simulink model "CurrentSource"  (R2024a)
settings: Solver=VariableStepAuto  StartTime=0.0  StopTime=10.0  RelTol=1e-3
undefined symbols (not defined in the file): b, R_B, Rsense, Vdd, Vpp, Vref
settings Model: Creator=Perij  LastModifiedBy=Perij

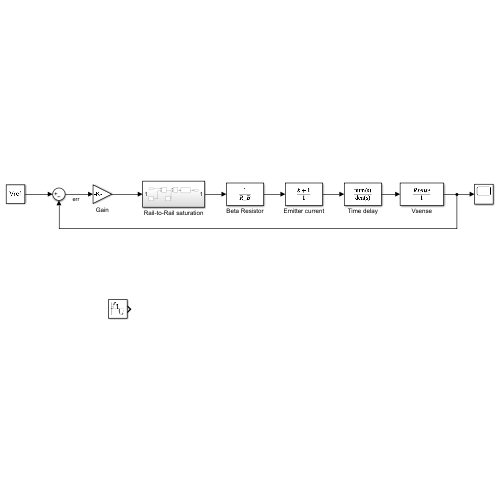
[thumbnail: Simulink's stored preview of the top-level diagram]
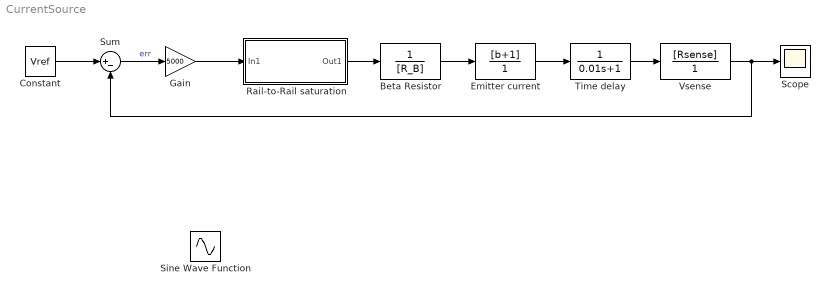
== system CurrentSource ==
  Beta Resistor : TransferFcn  Denominator=[R_B]
  Constant : Constant  Value=Vref
  Emitter current : TransferFcn  Numerator=[b+1]  Denominator=[1]
  Gain : Gain  Gain=5000
  Rail-to-Rail saturation : Subsystem
  Scope : Scope
  Sine Wave Function : Sin  Amplitude=20  Frequency=5  SampleTime=0.01
  Sum : Sum  Inputs=|+-
  Time delay : TransferFcn  Denominator=[0.01 1]
  Vsense : TransferFcn  Numerator=[Rsense]  Denominator=[1]
  wires:
  Rail-to-Rail saturation/1(Out1) -> Beta Resistor/1
  Constant/1 -> Sum/1
  Sum/1 -> Gain/1  "err"
  Gain/1 -> Rail-to-Rail saturation/1(In1)
  Beta Resistor/1 -> Emitter current/1
  Emitter current/1 -> Time delay/1
  Vsense/1 -> Sum/2, Scope/1
  Time delay/1 -> Vsense/1

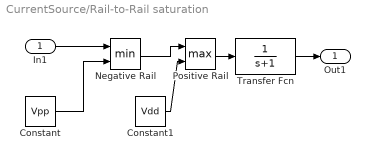
== system CurrentSource/Rail-to-Rail saturation ==
  In1 : Inport
  Constant : Constant  Value=Vpp
  Constant1 : Constant  Value=Vdd
  Negative Rail : MinMax  Inputs=2
  Positive Rail : MinMax  Function=max  Inputs=2
  Transfer Fcn : TransferFcn  Denominator=[1 1]
  Out1 : Outport
  wires:
  Negative Rail/1 -> Positive Rail/1
  In1/1 -> Negative Rail/1
  Positive Rail/1 -> Transfer Fcn/1
  Constant/1 -> Negative Rail/2
  Constant1/1 -> Positive Rail/2
  Transfer Fcn/1 -> Out1/1
